simulink model "plant"  (R2020a)
settings: Solver=VariableStepAuto  StartTime=0.0  StopTime=10.0  RelTol=1e-3
settings Model: Creator=Riyansh  LastModifiedBy=Riyansh

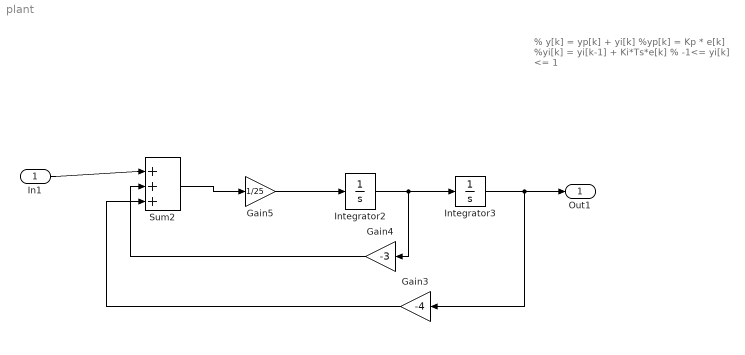
== system plant ==
  note: % y[k] = yp[k] + yi[k]
      |
      | %yp[k] = Kp * e[k]
      |
      | %yi[k] = yi[k-1] + Ki*Ts*e[k]
      |
      | % -1<= yi[k] <= 1
  In1 : Inport
  Gain3 : Gain  Gain=-4
  Gain4 : Gain  Gain=-3
  Gain5 : Gain  Gain=1/25
  Integrator2 : Integrator
  Integrator3 : Integrator
  Sum2 : Sum  Inputs=|+++
  Out1 : Outport
  wires:
  Sum2/1 -> Gain5/1
  Gain5/1 -> Integrator2/1
  Integrator2/1 -> Gain4/1, Integrator3/1
  Integrator3/1 -> Out1/1, Gain3/1
  Gain4/1 -> Sum2/2
  Gain3/1 -> Sum2/3
  In1/1 -> Sum2/1
